simulink library "VDIHeatExchanger"  (R2018b)
settings: Solver=ode45  StartTime=0.0  StopTime=10.0  RelTol=1e-3  EnableMultiTasking=on
undefined symbols (not defined in the file): path_carnot
libraries: carnot x2
settings Model: Creator=lena.frank  LastModifiedBy=drhf
settings DataIOCC: LimitDataPoints=on  SaveFormat=Array  SignalLoggingSaveFormat=ModelDataLogs
settings OptimizationCC: ExpressionDepthLimit=2147483647  LifeSpan=inf
settings DebuggingCC: UnderspecifiedInitializationDetection=Classic  MergeDetectMultiDrivingBlocksExec=none  SolverPrmCheckMsg=warning  FcnCallInpInsideContextMsg=warning  StateNameClashWarn=warning  SFUnexpectedBacktrackingDiag=warning  SFNoUnconditionalDefaultTransitionDiag=warning  SFExecutionAtInitializationDiag=none
settings HardwareCC: ProdBitPerPointer=32  ProdBitPerSizeT=32  ProdBitPerPtrDiffT=32  ProdLargestAtomicFloat=None  ProdIntDivRoundTo=Undefined  ProdEndianess=Unspecified  ProdWordSize=32  ProdHWDeviceType=32-bit Generic
settings ModelReferenceCC: PropagateSignalLabelsOutOfModel=off
settings SFSimCC: SimUseLocalCustomCode=off
settings RTWCC: RTWUseLocalCustomCode=off
settings CodeAppCC: StateflowObjectComments=on
settings GRTTargetCC: TargetLangStandard=C89/C90 (ANSI)  GeneratePreprocessorConditionals=Disable all  CombineOutputUpdateFcns=off  GRTInterface=on
settings ConfigComp: CovMetricSettings=dw  CovHtmlReporting=on  CovSaveCumulativeToWorkspaceVar=on  CovSaveSingleToWorkspaceVar=on  CovExternalEMLEnable=off

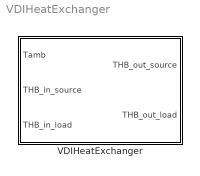
== system VDIHeatExchanger ==
  VDIHeatExchanger : Subsystem  mask(VDI heat exchanger){t0=20, PathName=fullfile(path_carnot('intlibsl'), 'Source', 'Heat_Exchanger', 'VDIHeatExchanger', 'parameter_set'), FileName='<user defined>', userPath=off, userParam=off, flowtype=1, a=0, b=0, c=0, d=0, ua0=2000, uahot=[0.04 0], uacold=[0.04 0], ualoss=3, cap=10e3, linh=20, quah=10, linc=20, quac=10}
      mask prompts: t0 "initial temperature [degree centigrade]"; PathName "Path"; FileName "Parameter set"; userPath "Edit path and name of parameter set"; userParam "User defined parameters"; flowtype "type of flow (0 = parallel, 0.5 = cross, 1 = counter)"; d "d (0.5 for symetric heat exchangers)"; ua0 "constant heat transfer ua0 [W/K]"; uahot "[mdot_nom_hot [kg/s] (>0) ,  ua_exp_hot (>=0)]"; uacold "[mdot_nom_cold [kg/s] (>0) ,  ua_exp_cold (>=0)]"; ualoss "heat losses to ambient [W/K]"; cap "capacity [J/K]"; linh "Source: pressure drop linear in massflow [Pa*s/kg]"; quah "Source: pressure drop quadratic in massflow [Pa*s²/kg²]"; linc "Load: pressure drop linear in massflow [Pa*s/kg]"; quac "Load: pressure drop quadratic in massflow [Pa*s²/kg²]"
      mask help:
      | Calculates the output THB of the hot and cold fluid of a heat exchanger.
      | The heat transfer is:
      | 	ua = ua0 * ( (mdot_hot/mdot_nom_hot)^ua_exp_hot
      |      	+ (mdot_cold/mdot_nom_cold)^ua_exp_cold )/2
      mask init:
      | flowtype = max(0, min(flowtype, 1));
      | linh = max(linh,0);
      | linc = max(linc,0);
      | quah = max(quah,0);
      | quac = max(quac,0);
      | uahot(1) = max(uahot(1), 1e-4);
      | uahot(2) = max(uahot(2), 0);
      | uacold(1) = max(uacold(1), 1e-4);
      | uacold(2) = max(uacold(2), 0);
      | cap = max(cap, 0.01);
      mask Help: web(fullfile(path_carnot('inthelp'),'VDIHeatExchanger.html'),'-helpbrowser')
      mask Callback userPath: [ok, param] = CarnotCallbacks_VDIHeatexchangerConf('UserEdit',gcbh);
      mask Callback userParam: [ok, param] = CarnotCallbacks_VDIHeatexchangerConf('UserEdit',gcbh);
      mask DialogControl Container14 Prompt: Calculation
      mask DialogControl ParameterGroupVar Prompt: Picking a parameter set
      mask DialogControl Control2 Prompt: Carnot public data
      mask DialogControl Control2 Callback: [ok, file] = CarnotCallbacks_VDIHeatexchangerConf('GetFilename',gcbh, 'public');
      mask DialogControl Control3 Prompt: Carnot internal data
      mask DialogControl Control3 Callback: [ok, file] = CarnotCallbacks_VDIHeatexchangerConf('GetFilename',gcbh, 'internal');
      mask DialogControl Control4 Prompt: Selected path
      mask DialogControl Control4 Callback: [ok, file] = CarnotCallbacks_VDIHeatexchangerConf('GetFilename',gcbh, 'selected');
      mask DialogControl ParameterTabVar0 Prompt: Thermal
      mask DialogControl Container9 Prompt: parameters for correction factor
      mask DialogControl ParameterTabVar01 Prompt: Hydraulic
      mask DialogControl Control5 Prompt: Save in Carnot internal data
      mask DialogControl Control5 Callback: [ok, param] = CarnotCallbacks_VDIHeatexchangerConf('SaveFilename',gcbh, 'internal','USTC');
      mask DialogControl Control6 Prompt: Save in selected path
      mask DialogControl Control6 Callback: [ok, param] = CarnotCallbacks_VDIHeatexchangerConf('SaveFilename',gcbh, 'selected','USTC');
      mask Display:
      | plot(-10,15,120,100,[40,70,70,40,40],[40 40 70 70 40],[55 55 62 48 55 55],[25 40 55 55 70 85],[30 40],[55 55],[70 80],[55 55])
      | disp('VDI')
      | port_label('input',1,'Ta')
      | port_label('input',2,'THBpri')
      | port_label('input',3,'THBsec')
      | port_label('output',1,'THBpri')
      | port_label('output',2,'THBsec')

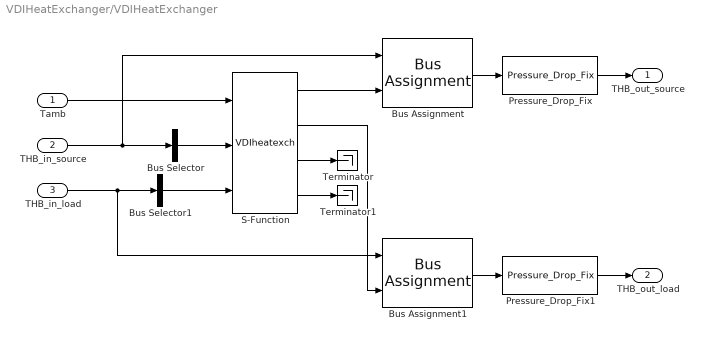
== system VDIHeatExchanger/VDIHeatExchanger ==
  Tamb : Inport
  THB_in_source : Inport  Port=2
  THB_in_load : Inport  Port=3
  Bus Assignment : BusAssignment  AssignedSignals=Temperature
  Bus Assignment1 : BusAssignment  AssignedSignals=Temperature
  Bus Selector : BusSelector  OutputSignals=Temperature,MassFlow,Pressure,FluidType,FluidMix  OutputAsBus=on
  Bus Selector1 : BusSelector  OutputSignals=Temperature,MassFlow,Pressure,FluidType,FluidMix  OutputAsBus=on
  Pressure_Drop_Fix : carnot/Basic/Pressure_Drop/Pressure_Drop_Fix  con=0  lin=linh  qua=quah
      settings: SourceProductName=Carnot
  Pressure_Drop_Fix1 : carnot/Basic/Pressure_Drop/Pressure_Drop_Fix  con=0  lin=linc  qua=quac
      settings: SourceProductName=Carnot
  S-Function : S-Function  FunctionName=VDIheatexch  Parameters=flowtype, ua0, uahot(1), uahot(2), uacold(1), uacold(2), ualoss, cap, t0,a,b,c,d  SFunctionDeploymentMode=off  EnableBusSupport=off
  Terminator : Terminator
  Terminator1 : Terminator
  THB_out_source : Outport
  THB_out_load : Outport  Port=2
  wires:
  Tamb/1 -> S-Function/1
  Bus Selector/1 -> S-Function/2
  S-Function/3 -> Terminator/1
  THB_in_source/1 -> Bus Selector/1, Bus Assignment/1
  THB_in_load/1 -> Bus Selector1/1, Bus Assignment1/1
  Bus Selector1/1 -> S-Function/3
  S-Function/1 -> Bus Assignment/2
  Bus Assignment/1 -> Pressure_Drop_Fix/1
  S-Function/2 -> Bus Assignment1/2
  Bus Assignment1/1 -> Pressure_Drop_Fix1/1
  Pressure_Drop_Fix/1 -> THB_out_source/1
  Pressure_Drop_Fix1/1 -> THB_out_load/1
  S-Function/4 -> Terminator1/1
